simulink model "tempModel"  (Simulink 7.9)
settings: Solver=ode45  StartTime=0.0  StopTime=100  RelTol=1e-6
values from neighbouring files (symbols this model uses):
  ti_auto = 2*kp*(tsx_auto - tnx_auto - tvx_auto)    [typeI_auto_tune_param_main.m]    (also in typeI_auto_tune_param_main_original.m)
  tp6 = plant_loc.tp6    [auto_tune_param_calculateOvs.m]    (also in auto_tune_param_calculateOvs_x_y.m; auto_tune_param_calculateOvs_x_y_margaris.m; auto_tune_param_main_ovsInvestigation_typeI.m = 0.01; auto_tune_param_main_pid.m)
  x_auto = tnx_auto + tvx_auto    (= 0)    [typeI_auto_tune_param_main.m]    (also in typeI_auto_tune_param_main_original.m)
  y_auto = plot_data_y(:,2)    [plotpaper.m]    (also in typeI_auto_tune_param_main.m = 0; typeI_auto_tune_param_main_original.m = 0)
libraries: cstblocks x5
settings Model: Creator=kostis  LastModifiedBy=kostis
settings OptimizationCC: InitFltsAndDblsToZero=on
settings DebuggingCC: FcnCallInpInsideContextMsg=Use local settings  StrictBusMsg=Warning
settings GRTTargetCC: CombineOutputUpdateFcns=off  GRTInterface=on

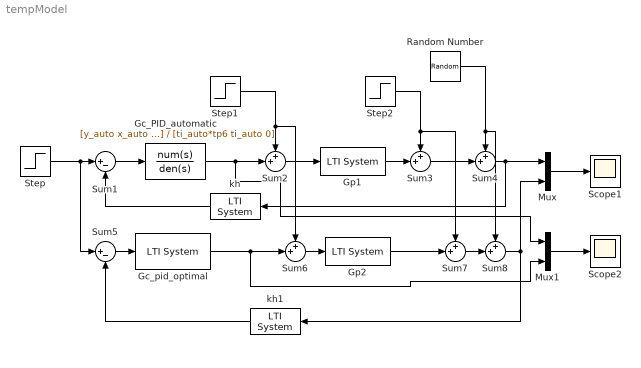
== system tempModel ==
  Gc_PID_automatic : TransferFcn  Numerator=[y_auto x_auto 1]  Denominator=[ti_auto*tp6 ti_auto 0]
  Gc_pid_optimal : cstblocks/LTI System  sys=Gc_pid_optimal  IC=[]
  Gp1 : cstblocks/LTI System  sys=Gp  IC=[]
  Gp2 : cstblocks/LTI System  sys=Gp  IC=[]
  Mux : Mux  Inputs=2
  Mux1 : Mux  Inputs=2
  Random Number : RandomNumber  Mean=0.000025  Variance=0.000025  Seed=0.00025  SampleTime=0.001
  Scope1 : Scope
      settings: YMin=0  YMax=2  SaveName=plot_data_y
  Scope2 : Scope
      settings: YMin=0  YMax=2  SaveName=plot_data_u
  Step : Step  Time=0  SampleTime=0
  Step1 : Step  Time=20  After=0.5  SampleTime=0
  Step2 : Step  Time=40  After=0.5  SampleTime=0
  Sum1 : Sum  Inputs=|+-
  Sum{2..4,6..8} (6 alike) : Sum  Inputs=++|
  Sum5 : Sum  Inputs=|+-
  kh : cstblocks/LTI System  sys=kh  IC=[]
  kh1 : cstblocks/LTI System  sys=kh  IC=[]
  wires:
  Sum1/1 -> Gc_PID_automatic/1
  kh/1 -> Sum1/2
  Mux/1 -> Scope1/1
  Step/1 -> Sum1/1, Sum5/1
  Gp1/1 -> Sum3/2
  Sum2/1 -> Gp1/1
  Gc_PID_automatic/1 -> Sum2/2, Mux1/1
  Step1/1 -> Sum2/1, Sum6/1
  Sum3/1 -> Sum4/2
  Sum4/1 -> Mux/1, kh/1
  Sum5/1 -> Gc_pid_optimal/1
  Gc_pid_optimal/1 -> Sum6/2, Mux1/2
  Sum6/1 -> Gp2/1
  Gp2/1 -> Sum7/2
  Step2/1 -> Sum3/1, Sum7/1
  kh1/1 -> Sum5/2
  Random Number/1 -> Sum4/1, Sum8/1
  Sum7/1 -> Sum8/2
  Sum8/1 -> kh1/1, Mux/2
  Mux1/1 -> Scope2/1
